simulink model "HW1no2"  (R2022b)
settings: Solver=VariableStepAuto  StartTime=0.0  StopTime=10.0  RelTol=1e-3
settings Model: Creator=mluser  LastModifiedBy=Lab417

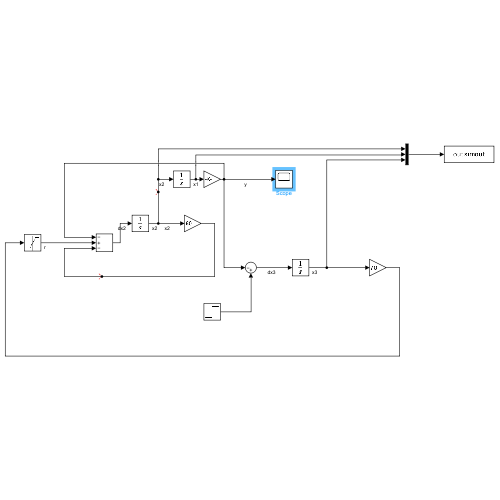
[thumbnail: Simulink's stored preview of the top-level diagram]
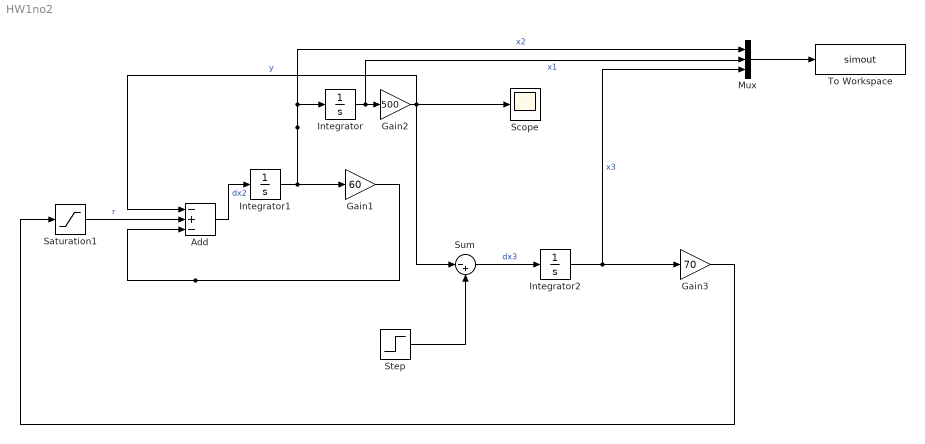
== system HW1no2 ==
  Add : Sum  Inputs=-+-
  Gain1 : Gain  Gain=60
  Gain2 : Gain  Gain=500
  Gain3 : Gain  Gain=70
  Integrator : Integrator
  Integrator1 : Integrator
  Integrator2 : Integrator
  Mux : Mux  Inputs=3
  Saturation1 : Saturate  UpperLimit=20  LowerLimit=-20
  Scope : Scope
  Step : Step  Time=0  SampleTime=0
  Sum : Sum  Inputs=|-+
  To Workspace : ToWorkspace  VariableName=simout  SaveFormat=Timeseries  SampleTime=-1
  wires:
  Integrator1/1 -> Gain1/1, Mux/1, Integrator/1  "x2"
  Add/1 -> Integrator1/1  "dx2"
  Gain1/1 -> Add/3
  Saturation1/1 -> Add/2  "r"
  Gain2/1 -> Scope/1, Add/1, Sum/1  "y"
  Gain3/1 -> Saturation1/1
  Sum/1 -> Integrator2/1  "dx3"
  Integrator2/1 -> Mux/3, Gain3/1  "x3"
  Integrator/1 -> Mux/2, Gain2/1  "x1"
  Step/1 -> Sum/2
  Mux/1 -> To Workspace/1
